simulink library "SEA_library_models"  (Simulink 8.6)
settings: Solver=ode45  StartTime=0.0  StopTime=10.0  RelTol=1e-3
undefined symbols (not defined in the file or in its folder): A, B, C
undefined symbols (not defined in the file): My_joint
libraries: simulink x7, cstblocks x4
settings Model: Creator=wesley  LastModifiedBy=wesley

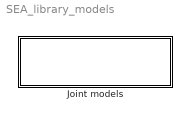
== system SEA_library_models ==
  Joint models : Subsystem

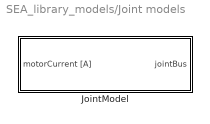
== system SEA_library_models/Joint models ==
  JointModel : Subsystem  mask{jointObj=My_joint, fc_vel=499, fc_torque=499, input_delay=0, output_delay=0, input_noise_enabled=off, output_noise_enabled=off, var_u=0.12^2, var_y=1.8e-10}
      mask prompts: jointObj "Joint Object"; fc_vel "Velocity filter cut-off frequency [Hz]"; fc_torque "Torque filter cut-off frequency [Hz]"; input_delay "Input delay (num samples)"; output_delay "Output delay (num samples)"; input_noise_enabled "Enable input noise"; output_noise_enabled "Enable measurement noise"; var_u "Input noise variance"; var_y "Measurement noise variance"
      mask init:
      | % Get linear dynamics matrices
      | [A, B, C, I, D, K] = jointObj.getDynamicsMatrices();
      | 
      | handleMatlabFunctionBlock(gcb,jointObj);
      | 
      | % % Other properties
      | Ts = jointObj.Ts;
      | k_t = jointObj.k_t;
      | k_b = jointObj.k_b;
      | 
      | % If noise is disabled, overwrite the given variances
      | if (input_noise_enabled == 0)
      |     var_u = 0;
      | end
      | if (output_noise_enabled == 0)
      | 	var_y = 0;
      | end
      | % 
      | % % ---------------------------------
      | % % Edit contents of nonLinDynamicsFcn block
      | % % ---------------------------------
      | % thisBlock = gcb;
      | % funName = 'nonLinDynamicsFcn';
      | % fcnBlock = [thisBlock, '/', funName];
      | % intBlock = [thisBlock, '/', 'Integrator'];
      | % sumBlock = [thisBlock, '/', 'Sum'];
      | % %refBlock = get_param(fcnBlock,'ReferenceBlock');
      | % 
      | % % Locate the property, which stores the source code text
      | % % r = slroot;
      | % %  scriptBlock = r.find('-isa','Stateflow.EMChart','path',fcnBlock);
      | % r = slroot;
      | % scriptBlock = r.find('-isa','Stateflow.EMChart','path',fcnBlock);
      | % if isempty(scriptBlock)
      | %     load_system('simulink');
      | %     add_block('simulink/User-Defined Functions/MATLAB Function',fcnBlock,...
      | %         'Position', [630 312 700 358],...
      | %         'Orientation', 'left');
      | %     add_line(thisBlock,[funName '/1'], ['Sum/1'],'AutoRouting','On');
      | %     add_line(thisBlock,[funName '/1'], ['nonLinearDynamicsScope/1'],'AutoRouting','On');
      | %     add_line(thisBlock,'Integrator/1',[funName '/1'],'AutoRouting','On')
      | %     
      | %     scriptBlock = r.find('-isa','Stateflow.EMChart','path',fcnBlock);
      | %     if isempty(scriptBlock)
      | %         error(message('symbolic:sym:matlabFunctionBlock:CouldNotCreate', fcnBlock));
      | %     end
      | % end
      | % if size(scriptBlock) > 1
      | %     error(message('symbolic:sym:matlabFunctionBlock:AmbiguousBlock', fcnBlock));
      | % end
      | % if ~isa(scriptBlock,'Stateflow.EMChart')
      | %     error(message('symbolic:sym:matlabFunctionBlock:InvalidBlock', fcnBlock));
      | % end
      | %  
      | %  
      | % % The strategy is to write a temporary text file to format the code.
      | % % Then read the file again and paste the string into the source code
      | % % property.
      | % file = 'nonLinDynamicsFcnTMP.m';
      | % fid = fopen(file,'wt+');
      | % tmp = onCleanup(@()delete(file)); % file guard -> removes temporary file upon crash.
      | % 
      | % fprintf(fid,'%s\n',['function tau = nonLinDynamics(x)']);   % write signature
      | % fprintf(fid,'%s\n\n',['%#codegen']);                            % indicate possibility of code generation
      | % 
      | % % Make parameters available inside the function
      | % s = jointObj.getParams();   % Get params struct
      | % fields = fieldnames(s)';    % Get fieldnames
      | % N = numel(fields);          % Loop through all fields and print
      | % for i=1:N
      | %     val = s.(fields{i});
      | %     if (isnumeric(val))
      | %         % Numeric values
      | %         fprintf(fid, 'params.%s = %f;\n', fields{i}, s.(fields{i}));
      | %     elseif (iscell(val))
      | %         % String cells
      | %         fprintf(fid, '%%params.%s = {', fields{i});
      | %         for j=1:length(val)
      | %             fprintf(fid, '''%s''', s.(fields{i}){j});
      | %             if (j < length(val))
      | %                 fprintf(fid, ', ');
      | %             end
      | %         end
      | %         fprintf(fid, '}; %% Cell arrays are not supported for code generation.\n');
      | %     else
      | %         % Strings
      | %         fprintf(fid, 'params.%s = ''%s'';\n', fields{i}, s.(fields{i}));
      | %     end
      | % end
      | % 
      | % % Write the nonlinear model code
      | % argStr = '(params,x)';
      | % nonlinearModelName = jointObj.nonLinearModelName;
      | % nonlinearModelName_multiple = 0;
      | % if (iscell(nonlinearModelName) && length(nonlinearModelName) > 1)
      | %     nonlinearModelName_multiple = 1;
      | % end
      | % 
      | % fStr = '';
      | % if (~isempty(nonlinearModelName) && nonlinearModelName_multiple)
      | %     % Multiple nonlinear terms
      | %     for i=1:length(nonlinearModelName)
      | %         fStr = strcat(fStr, nonlinearModelName(i), argStr);
      | %         if (i < length(nonlinearModelName))
      | %             fStr = strcat(fStr, char(' + '));
      | %         end
      | %     end
      | % elseif ~isempty(nonlinearModelName)
      | %     % Single nonlinear term
      | %     fStr = strcat(nonlinearModelName,argStr);
      | % else
      | %     % No nonlinear terms
      | %     fStr = sprintf('%s',  'zeros(size(x))');
      | % end
      | % fStr = strcat('tau = ', fStr, ';');
      | % fprintf(fid, '%s\n', char(fStr));
      | % 
      | % % End methods
      | % fprintf(fid,'\tend\n\n');
      | % 
      | % 
      | % contents = fileread(file);
      | % scriptBlock.Script = sprintf('%s\n',contents);
      | % save_system
      | % sfsave
      | % 
      | % fclose(fid);
      | % clear('tmp');
      | % 
      | % outPortAddress = [fcnBlock, '/', 'tau'];
      | % set_param(outPortAddress,'PortDimensions',num2str(size(A,1)));
      | %
      settings: ModelCloseFcn=sfsave  DestroyFcn=sfsave
      mask Callback input_noise_enabled: toggleMaskFields(gcbh, 'input_noise_enabled', 'var_u');
      mask Callback output_noise_enabled: toggleMaskFields(gcbh, 'output_noise_enabled', 'var_y');

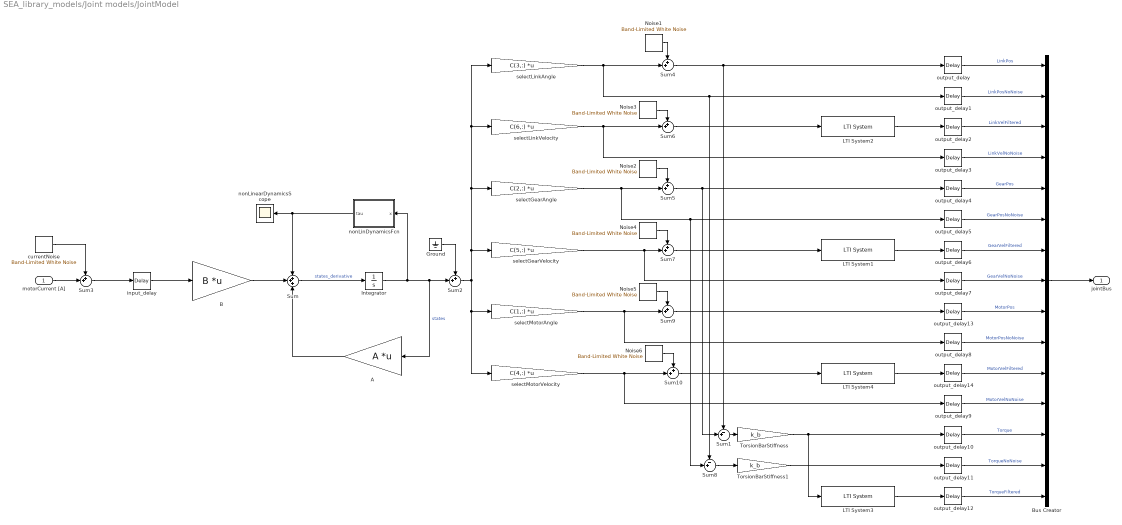
== system SEA_library_models/Joint models/JointModel ==
  motorCurrent [A] : Inport
  A : Gain  Gain=A  Multiplication=Matrix(K*u)
  B : Gain  Gain=B  Multiplication=Matrix(K*u)
  Bus Creator : BusCreator  Inputs=15
  Ground : Ground
  Integrator : Integrator
  LTI System1 : cstblocks/LTI System  sys=c2d(tf([2*pi*fc_vel],[1 2*pi*fc_vel]),Ts)  IC=[]
  LTI System2 : cstblocks/LTI System  sys=c2d(tf([2*pi*fc_vel],[1 2*pi*fc_vel]),Ts)  IC=[]
  LTI System3 : cstblocks/LTI System  sys=c2d(tf([2*pi*fc_torque],[1 2*pi*fc_torque]),Ts)  IC=[]
  LTI System4 : cstblocks/LTI System  sys=c2d(tf([2*pi*fc_vel],[1 2*pi*fc_vel]),Ts)  IC=[]
  Noise1 : simulink/Sources/Band-Limited White Noise  Cov=var_y * Ts  Ts=Ts  seed=[3846513]
  Noise2 : simulink/Sources/Band-Limited White Noise  Cov=var_y * Ts  Ts=Ts  seed=[11563454]
  Noise3 : simulink/Sources/Band-Limited White Noise  Cov=(var_y * Ts) * (2/Ts^2)  Ts=Ts  seed=[982379842]
  Noise4 : simulink/Sources/Band-Limited White Noise  Cov=(var_y * Ts) * (2/Ts^2)  Ts=Ts  seed=[3249879708]
  Noise5 : simulink/Sources/Band-Limited White Noise  Cov=var_y * Ts  Ts=Ts  seed=[24326]
  Noise6 : simulink/Sources/Band-Limited White Noise  Cov=(var_y * Ts) * (2/Ts^2)  Ts=Ts  seed=[2134245675]
  Sum : Sum  Inputs=+++
  Sum1 : Sum  Inputs=-+|
  Sum{2..7,9..10} (8 alike) : Sum  Inputs=++|
  Sum8 : Sum  Inputs=-+|
  TorsionBarStiffness : Gain  Gain=k_b
  TorsionBarStiffness1 : Gain  Gain=k_b
  currentNoise : simulink/Sources/Band-Limited White Noise  Cov=var_u * Ts  Ts=Ts  seed=[2435345645]
  input_delay : TransportDelay  DelayTime=input_delay * jointObj.Ts  TransDelayFeedthrough=on
  nonLinDynamicsFcn : MATLAB Function  TreatAsAtomicUnit=on
  nonLinearDynamicsScope : Scope
  output_delay{,1..14} (15 alike) : TransportDelay  DelayTime=output_delay * jointObj.Ts
  selectGearAngle : Gain  Gain=C(2,:)  Multiplication=Matrix(K*u)
  selectGearVelocity : Gain  Gain=C(5,:)  Multiplication=Matrix(K*u)
  selectLinkAngle : Gain  Gain=C(3,:)  Multiplication=Matrix(K*u)
  selectLinkVelocity : Gain  Gain=C(6,:)  Multiplication=Matrix(K*u)
  selectMotorAngle : Gain  Gain=C(1,:)  Multiplication=Matrix(K*u)
  selectMotorVelocity : Gain  Gain=C(4,:)  Multiplication=Matrix(K*u)
  jointBus : Outport
  wires:
  nonLinDynamicsFcn/1(tau) -> nonLinearDynamicsScope/1, Sum/1
  Bus Creator/1 -> jointBus/1
  input_delay/1 -> B/1
  Sum3/1 -> input_delay/1
  TorsionBarStiffness1/1 -> output_delay11/1
  selectGearAngle/1 -> Sum5/2, output_delay5/1, Sum8/2
  Sum8/1 -> TorsionBarStiffness1/1
  Sum7/1 -> LTI System1/1
  Noise4/1 -> Sum7/1
  Noise3/1 -> Sum6/1
  Sum6/1 -> LTI System2/1
  currentNoise/1 -> Sum3/1
  Noise2/1 -> Sum5/1
  Noise1/1 -> Sum4/1
  selectLinkAngle/1 -> Sum4/2, output_delay1/1, Sum8/1
  Sum4/1 -> output_delay/1, Sum1/1
  selectMotorVelocity/1 -> output_delay9/1, Sum10/2
  LTI System1/1 -> output_delay6/1
  selectGearVelocity/1 -> Sum7/2, output_delay7/1
  Sum/1 -> Integrator/1  "states_derivative"
  LTI System3/1 -> output_delay12/1
  Sum5/1 -> output_delay4/1, Sum1/2
  TorsionBarStiffness/1 -> LTI System3/1, output_delay10/1
  selectMotorAngle/1 -> output_delay8/1, Sum9/2
  selectLinkVelocity/1 -> Sum6/2, output_delay3/1
  LTI System2/1 -> output_delay2/1
  motorCurrent [A]/1 -> Sum3/2
  Sum1/1 -> TorsionBarStiffness/1
  Integrator/1 -> nonLinDynamicsFcn/1(x), Sum2/2, A/1  "states"
  Sum2/1 -> selectMotorVelocity/1, selectMotorAngle/1, selectGearAngle/1, selectLinkVelocity/1, selectLinkAngle/1, selectGearVelocity/1
  Ground/1 -> Sum2/1
  B/1 -> Sum/2
  A/1 -> Sum/3
  output_delay/1 -> Bus Creator/1  "LinkPos"
  output_delay1/1 -> Bus Creator/2  "LinkPosNoNoise"
  output_delay2/1 -> Bus Creator/3  "LinkVelFiltered"
  output_delay3/1 -> Bus Creator/4  "LinkVelNoNoise"
  output_delay4/1 -> Bus Creator/5  "GearPos"
  output_delay5/1 -> Bus Creator/6  "GearPosNoNoise"
  output_delay6/1 -> Bus Creator/7  "GearVelFiltered"
  output_delay7/1 -> Bus Creator/8  "GearVelNoNoise"
  output_delay8/1 -> Bus Creator/10  "MotorPosNoNoise"
  output_delay9/1 -> Bus Creator/12  "MotorVelNoNoise"
  output_delay10/1 -> Bus Creator/13  "Torque"
  output_delay11/1 -> Bus Creator/14  "TorqueNoNoise"
  output_delay12/1 -> Bus Creator/15  "TorqueFiltered"
  Noise5/1 -> Sum9/1
  Sum9/1 -> output_delay13/1
  LTI System4/1 -> output_delay14/1
  output_delay13/1 -> Bus Creator/9  "MotorPos"
  output_delay14/1 -> Bus Creator/11  "MotorVelFiltered"
  Noise6/1 -> Sum10/1
  Sum10/1 -> LTI System4/1

== matlab function Joint models/JointModel/nonLinDynamicsFcn ==
  data: x input double; tau output double
function tau = nonLinDynamics(x)
%#codegen

params.verbose = 0.000000;
params.debug = 0.000000;
params.I_m = 0.854775;
params.I_g = 0.569827;
params.I_b = 0.055500;
params.k_g = 31000.000000;
params.k_b = 2800.000000;
params.d_m = 6.000000;
params.d_g = 6.000000;
params.d_b = 7.000000;
params.d_m_n = 5.000000;
params.d_g_n = 5.000000;
params.d_b_n = 5.000000;
params.d_mg = 144.000000;
params.d_gb = 2.000000;
params.d_cm = 0.676650;
params.d_cg = 0.676650;
params.d_cb = 0.000000;
params.d_cm_n = 0.502900;
params.d_cg_n = 0.502900;
params.d_cb_n = 0.000000;
params.n = 80.000000;
params.k_t = 0.045500;
params.r = 0.099000;
params.x = 0.000000;
params.Ts = 0.001000;
params.name = 'WMBig_TestRig_continuous_output_fixed';
params.paramName = 'WMBig_TestRig';
params.modelName = 'continuous_output_fixed';
params.nonlinearModelName = '';
tau =zeros(size(x));
	end
